simulink model "zt"  (Simulink 7.3)
settings: Solver=ode3  StartTime=0.0  StopTime=10.0  FixedStep=1  RelTol=1e-3
settings Model: Creator=hnine  LastModifiedBy=hnine
settings OptimizationCC: InitFltsAndDblsToZero=on
settings DebuggingCC: SaveWithParameterizedLinksMsg=none
settings GRTTargetCC: TargetFcnLib=ansi_tfl_tmw.mat

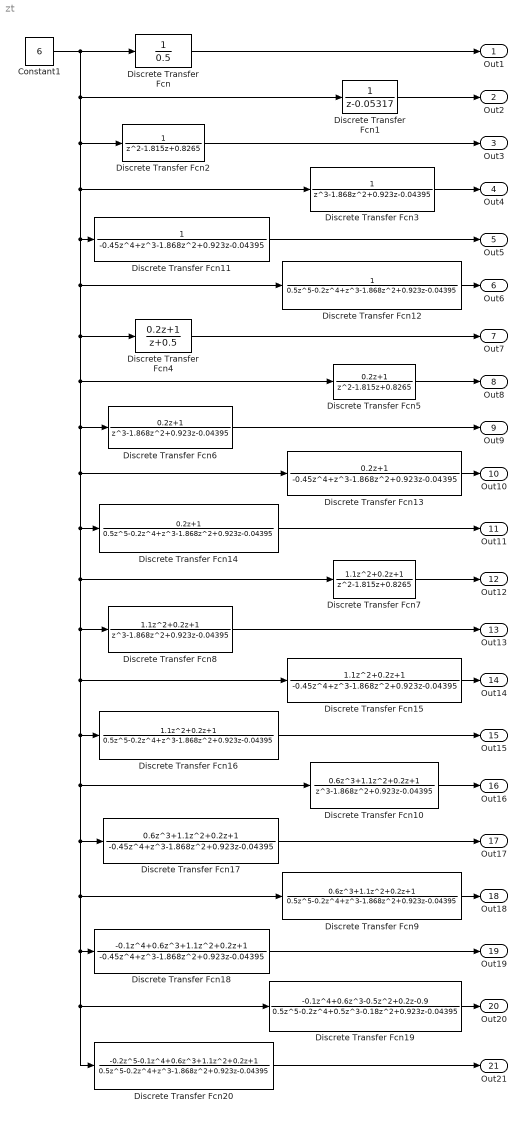
== system zt ==
  Constant1 : Constant  Value=6  OutDataTypeMode=double  OutDataType=sfix(16)  OutScaling=2^0  OutDataTypeStr=double
  Discrete Transfer Fcn : DiscreteTransferFcn  Denominator=[0.5]
  Discrete Transfer Fcn1 : DiscreteTransferFcn  Denominator=[1 -0.05317]
  Discrete Transfer Fcn10 : DiscreteTransferFcn  Numerator=[0.6 1.1 0.2 1]  Denominator=[1 -1.868 0.923 -0.04395]
  Discrete Transfer Fcn11 : DiscreteTransferFcn  Denominator=[-0.45 1 -1.868 0.923 -0.04395]
  Discrete Transfer Fcn12 : DiscreteTransferFcn  Denominator=[0.5 -0.2 1 -1.868 0.923 -0.04395]
  Discrete Transfer Fcn13 : DiscreteTransferFcn  Numerator=[0.2 1]  Denominator=[-0.45 1 -1.868 0.923 -0.04395]
  Discrete Transfer Fcn14 : DiscreteTransferFcn  Numerator=[0.2 1]  Denominator=[0.5 -0.2 1 -1.868 0.923 -0.04395]
  Discrete Transfer Fcn15 : DiscreteTransferFcn  Numerator=[1.1 0.2 1]  Denominator=[-0.45 1 -1.868 0.923 -0.04395]
  Discrete Transfer Fcn16 : DiscreteTransferFcn  Numerator=[1.1 0.2 1]  Denominator=[0.5 -0.2 1 -1.868 0.923 -0.04395]
  Discrete Transfer Fcn17 : DiscreteTransferFcn  Numerator=[0.6 1.1 0.2 1]  Denominator=[-0.45 1 -1.868 0.923 -0.04395]
  Discrete Transfer Fcn18 : DiscreteTransferFcn  Numerator=[-0.1 0.6 1.1 0.2 1]  Denominator=[-0.45 1 -1.868 0.923 -0.04395]
  Discrete Transfer Fcn19 : DiscreteTransferFcn  Numerator=[-0.1 0.6 -0.5 0.2 -0.9]  Denominator=[0.5 -0.2 0.5 -0.18 0.923 -0.04395]
  Discrete Transfer Fcn2 : DiscreteTransferFcn  Denominator=[1 -1.815 0.8265]
  Discrete Transfer Fcn20 : DiscreteTransferFcn  Numerator=[-0.2 -0.1 0.6 1.1 0.2 1]  Denominator=[0.5 -0.2 1 -1.868 0.923 -0.04395]
  Discrete Transfer Fcn3 : DiscreteTransferFcn  Denominator=[1 -1.868 0.923 -0.04395]
  Discrete Transfer Fcn4 : DiscreteTransferFcn  Numerator=[0.2 1]
  Discrete Transfer Fcn5 : DiscreteTransferFcn  Numerator=[0.2 1]  Denominator=[1 -1.815 0.8265]
  Discrete Transfer Fcn6 : DiscreteTransferFcn  Numerator=[0.2 1]  Denominator=[1 -1.868 0.923 -0.04395]
  Discrete Transfer Fcn7 : DiscreteTransferFcn  Numerator=[1.1 0.2 1]  Denominator=[1 -1.815 0.8265]
  Discrete Transfer Fcn8 : DiscreteTransferFcn  Numerator=[1.1 0.2 1]  Denominator=[1 -1.868 0.923 -0.04395]
  Discrete Transfer Fcn9 : DiscreteTransferFcn  Numerator=[0.6 1.1 0.2 1]  Denominator=[0.5 -0.2 1 -1.868 0.923 -0.04395]
  Out1 : Outport  OutDataType=sfix(16)  OutScaling=2^0
  Out2 : Outport  Port=2  OutDataType=sfix(16)  OutScaling=2^0
  Out3 : Outport  Port=3  OutDataType=sfix(16)  OutScaling=2^0
  Out4 : Outport  Port=4  OutDataType=sfix(16)  OutScaling=2^0
  Out5 : Outport  Port=5  OutDataType=sfix(16)  OutScaling=2^0
  Out6 : Outport  Port=6  OutDataType=sfix(16)  OutScaling=2^0
  Out7 : Outport  Port=7  OutDataType=sfix(16)  OutScaling=2^0
  Out8 : Outport  Port=8  OutDataType=sfix(16)  OutScaling=2^0
  Out9 : Outport  Port=9  OutDataType=sfix(16)  OutScaling=2^0
  Out10 : Outport  Port=10  OutDataType=sfix(16)  OutScaling=2^0
  Out11 : Outport  Port=11  OutDataType=sfix(16)  OutScaling=2^0
  Out12 : Outport  Port=12  OutDataType=sfix(16)  OutScaling=2^0
  Out13 : Outport  Port=13  OutDataType=sfix(16)  OutScaling=2^0
  Out14 : Outport  Port=14  OutDataType=sfix(16)  OutScaling=2^0
  Out15 : Outport  Port=15  OutDataType=sfix(16)  OutScaling=2^0
  Out16 : Outport  Port=16  OutDataType=sfix(16)  OutScaling=2^0
  Out17 : Outport  Port=17  OutDataType=sfix(16)  OutScaling=2^0
  Out18 : Outport  Port=18  OutDataType=sfix(16)  OutScaling=2^0
  Out19 : Outport  Port=19  OutDataType=sfix(16)  OutScaling=2^0
  Out20 : Outport  Port=20  OutDataType=sfix(16)  OutScaling=2^0
  Out21 : Outport  Port=21  OutDataType=sfix(16)  OutScaling=2^0
  wires:
  Constant1/1 -> Discrete Transfer Fcn/1, Discrete Transfer Fcn1/1, Discrete Transfer Fcn2/1, Discrete Transfer Fcn3/1, Discrete Transfer Fcn4/1, Discrete Transfer Fcn5/1, Discrete Transfer Fcn6/1, Discrete Transfer Fcn13/1, Discrete Transfer Fcn8/1, Discrete Transfer Fcn15/1, Discrete Transfer Fcn16/1, Discrete Transfer Fcn10/1, Discrete Transfer Fcn17/1, Discrete Transfer Fcn9/1, Discrete Transfer Fcn18/1, Discrete Transfer Fcn19/1, Discrete Transfer Fcn20/1, Discrete Transfer Fcn7/1, Discrete Transfer Fcn14/1, Discrete Transfer Fcn12/1, Discrete Transfer Fcn11/1
  Discrete Transfer Fcn/1 -> Out1/1
  Discrete Transfer Fcn1/1 -> Out2/1
  Discrete Transfer Fcn2/1 -> Out3/1
  Discrete Transfer Fcn3/1 -> Out4/1
  Discrete Transfer Fcn4/1 -> Out7/1
  Discrete Transfer Fcn5/1 -> Out8/1
  Discrete Transfer Fcn6/1 -> Out9/1
  Discrete Transfer Fcn7/1 -> Out12/1
  Discrete Transfer Fcn8/1 -> Out13/1
  Discrete Transfer Fcn11/1 -> Out5/1
  Discrete Transfer Fcn12/1 -> Out6/1
  Discrete Transfer Fcn13/1 -> Out10/1
  Discrete Transfer Fcn14/1 -> Out11/1
  Discrete Transfer Fcn15/1 -> Out14/1
  Discrete Transfer Fcn16/1 -> Out15/1
  Discrete Transfer Fcn10/1 -> Out16/1
  Discrete Transfer Fcn17/1 -> Out17/1
  Discrete Transfer Fcn9/1 -> Out18/1
  Discrete Transfer Fcn18/1 -> Out19/1
  Discrete Transfer Fcn19/1 -> Out20/1
  Discrete Transfer Fcn20/1 -> Out21/1
